simulink model "MagnetoShield_Calibration"  (R2019a)
settings: Solver=FixedStepAuto  StartTime=0.0  StopTime=10  RelTol=1e-3  EnableMultiTasking=on
libraries: arduinolib x1
settings Model: SimulationMode=external  ExtModeTrigDuration=2  Creator=Jakub  LastModifiedBy=Gergely
settings OptimizationCC: EnhancedBackFolding=on  PassReuseOutputArgsAs=Individual arguments  MaxStackSize=64  OptimizeBlockOrder=speed  DifferentSizesBufferReuse=on  OptimizationCustomize=off
settings DebuggingCC: ParameterTunabilityLossMsg=error
settings HardwareCC: ProdBitPerPointer=32  ProdBitPerSizeT=32  ProdBitPerPtrDiffT=32  ProdLargestAtomicInteger=Long  ProdLargestAtomicFloat=Double  ProdWordSize=32  ProdHWDeviceType=ARM Compatible->ARM Cortex
settings SFSimCC: MATLABDynamicMemAlloc=off
settings RTWCC: SystemTargetFile=ert.tlc  HardwareBoard=Arduino Due  TLCOptions=-aInlineSetEventsForThisBaseRateFcn=TLC_FALSE -aSuppressMultiTaskScheduler=TLC_FALSE -aRateBasedStepFcn=1  TemplateMakefile=ert_default_tmf  GenerateReport=on  Toolchain=Arduino ARM  BuildConfiguration=Faster Runs  IncludeHyperlinkInReport=on  LaunchReport=on  GenerateTraceInfo=on  GenerateTraceReport=on  GenerateTraceReportSl=on  GenerateTraceReportSf=on  GenerateTraceReportEml=on
settings CodeAppCC: ForceParamTrailComments=on  IgnoreCustomStorageClasses=off  OperatorAnnotations=on  SimulinkDataObjDesc=on  SFDataObjDesc=on  InsertBlockDesc=on
settings ERTTargetCC: SupportContinuousTime=on  SupportVariableSizeSignals=on  ExtModeStaticAllocSize=24576

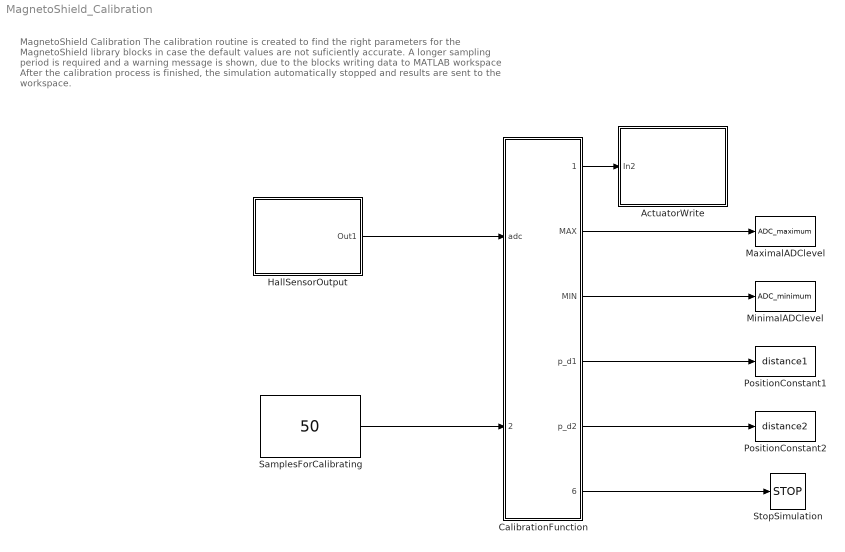
== system MagnetoShield_Calibration ==
  note: MagnetoShield Calibration
      | The calibration routine is created to find the right parameters for the MagnetoShield library blocks in case the default values are not suficiently accurate.
      |
      | A longer sampling period is required and a warning message is shown, due to the blocks writing data to MATLAB workspace
      |
      | After the calibration process is finished, the simulation automatically stopped and results are sent to the workspace.
  ActuatorWrite : Subsystem  AncestorBlock=MagnetoLibrary/ActuatoWrite  mask{Board=DUE, Units=Volts}
      mask prompts: Board "Type of the Arduino board"; Units "Input unite"
      mask help:
      | ActuatorWrite block allows to set desired voltage value on the electromagnet. The desired value can be expresed as voltage, percentage of maximal possible voltage or as a value of the magnetic field in Gausses as well.
      | This block converts input control signal into suficient form (16-bit number) and writes the information on the MCP4725-DAC converter.
      | Maximal voltage range: 0-12 V
      mask init:
      | mask_popup = get_param(gcb,'Board'); % which popup is choosen
      | % path to the I2C Write block
      | system = gcb;
      | way = strcat(system,'/I2C Write UNO');
      | % set Module based on Arduino type
      | if strcmp(mask_popup(1),'U')
      |     set_param(way,'I2CModule','0'); % Uno/Mega - module 0
      | elseif strcmp(mask_popup(1),'D')
      |     set_param(way,'I2CModule','1'); % Due - module 1
      | end
      settings: CopyFcn=set_param(gcb, 'LinkStatus', 'inactive')
      mask TypeOptions Board: UNO/MEGA | DUE
      mask TypeOptions Units: Volts | Percents | DAC levels
      mask DialogControl DescGroupVar Prompt: ActuatorWrite block
      mask Display: image('assets\MagnetoFig\ActuatorWrite.bmp');
  CalibrationFunction : MATLAB Function  TreatAsAtomicUnit=on
  HallSensorOutput : Subsystem  AncestorBlock=MagnetoLibrary/MagnetoShieldPins  mask{PIN=Hall sensor pin (A3), sampling=0.008}
      mask prompts: PIN "Choose pin"; sampling "Sampling period [s]"
      mask help:
      | User can choose a pin on which the data should be processed.
      | >Hall sensor pin - data about the possition of the levitating magnet.
      | >Voltage pin - voltage on the electromagnet
      | >Current pin - current crossing the electromagnet
      | >Reference pin - data from potentiometer, used as adjustable analog reference
      | (output = double)
      mask init:
      | letter = PIN;
      | if letter==1
      | path='assets\MagnetoFig\Pins\hpin.bmp';
      | elseif letter==2
      | path='assets\MagnetoFig\Pins\vpin.bmp';
      | elseif letter==3
      | path='assets\MagnetoFig\Pins\cpin.bmp';
      | else
      | path='assets\MagnetoFig\Pins\ppin.bmp';    
      | end
      settings: CopyFcn=set_param(gcb, 'LinkStatus', 'inactive')
      mask TypeOptions PIN: Hall sensor pin (A3) | Voltage pin (A1) | Current pin (A2) | Reference pin (A0)
      mask Callback PIN:
      | mask_popup = get_param(gcb,'PIN'); % which popup is choosen
      | % path to the I2C Write block
      | system = gcb;
      | way = strcat(system,'/Analog Input');
      | % set Module based on Arduino type
      | if strcmp(mask_popup(1),'H')
      |     set_param(way,'pinNumber','3'); % Uno/Mega - module 0
      | elseif strcmp(mask_popup(1),'V')
      |     set_param(way,'pinNumber','1'); % Due - module 1
      | elseif strcmp(mask_popup(1),'C')
      |     set_param(way,'pinNumber','2'); % Due - module 1
      | elseif strcmp(mask_popup(1),'R')
      |     set_param(way,'pinNumber','0'); % Due - module 11
      | end
      mask DialogControl DescGroupVar Prompt: MagnetoShieldPins block
      mask Display: image(path);
  MaximalADClevel : ToWorkspace  VariableName=ADC_maximum  SampleTime=-1
      settings: MaxDataPoints=1  Save2DSignal=2-D array (concatenate along first dimension)
  MinimalADClevel : ToWorkspace  VariableName=ADC_minimum  SampleTime=-1
      settings: MaxDataPoints=1  Save2DSignal=2-D array (concatenate along first dimension)
  PositionConstant1 : ToWorkspace  VariableName=distance1  SampleTime=-1
      settings: MaxDataPoints=1  Save2DSignal=2-D array (concatenate along first dimension)
  PositionConstant2 : ToWorkspace  VariableName=distance2  SampleTime=-1
      settings: MaxDataPoints=1  Save2DSignal=2-D array (concatenate along first dimension)
  SamplesForCalibrating : Constant  Value=50  SampleTime=0.008
  StopSimulation : Stop
  wires:
  CalibrationFunction/1(voltage) -> ActuatorWrite/1(In2)
  CalibrationFunction/2(MAX) -> MaximalADClevel/1
  CalibrationFunction/3(MIN) -> MinimalADClevel/1
  CalibrationFunction/6(terminate) -> StopSimulation/1
  HallSensorOutput/1(Out1) -> CalibrationFunction/1(adc)
  SamplesForCalibrating/1 -> CalibrationFunction/2(samples)
  CalibrationFunction/4(p_d1) -> PositionConstant1/1
  CalibrationFunction/5(p_d2) -> PositionConstant2/1

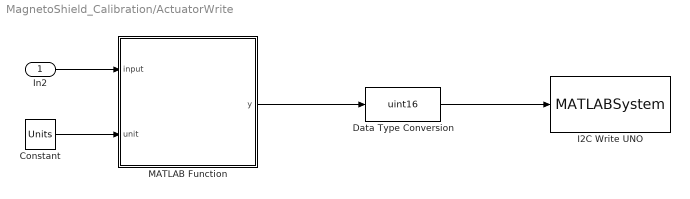
== system MagnetoShield_Calibration/ActuatorWrite ==
  In2 : Inport
  Constant : Constant  Value=Units
  Data Type Conversion : DataTypeConversion  OutDataTypeStr=uint16
  I2C Write UNO : MATLABSystem  AncestorBlock=arduinolib/I2C Write  InitFcn=|  System=codertarget.arduinobase.internal.arduinoI2CWrite  I2CModule=1  Mode=Master  SlaveAddress=96  SlaveByteOrder=BigEndian  Direction=Transmitter  RegisterAddressMode=off  RegisterAddress=0  SlaveDataType=uint8  DataLength=1  NoAck=off  RepeatedStart=off  OutputStatus=off  blockPlatform=ARDUINO
      | codertarget.arduinobase.blocks.registerI2CBlock(gcbh);
      | codertarget.arduinobase.blocks.arduinoBlockInitFcnCallback(gcbh);
      mask Type: I2C Write
      mask Display:
      | color('white');
      | plot([100,100,100,100],[100,100,100,100]);
      | plot([0,0,0,0],[0,0,0,0]);
      | color('blue');
      | text(99, 92, 'ARDUINO', 'horizontalAlignment', 'right');
      | color('black');
      | text(50,60,'\fontsize{12}\bfI2C','texmode','on','horizontalAlignment','center','verticalAlignment','middle');
      | text(50,40,'\fontsize{10}\bfMaster Write','texmode','on','horizontalAlignment','center','verticalAlignment','middle');
      | text(50,15,'Slave: 0x60' ,'horizontalAlignment', 'center');
      | port_label('input',1,'Data');
  MATLAB Function : MATLAB Function  TreatAsAtomicUnit=on
  wires:
  MATLAB Function/1(y) -> Data Type Conversion/1
  Data Type Conversion/1 -> I2C Write UNO/1
  Constant/1 -> MATLAB Function/2(unit)
  In2/1 -> MATLAB Function/1(input)

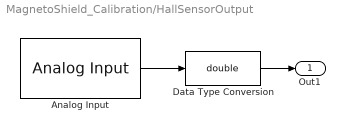
== system MagnetoShield_Calibration/HallSensorOutput ==
  Analog Input : arduinolib/Analog Input  pinNumber=3  ReadResultsOnly=off  ConversionTriggerSource=Software  ExternalTriggerType=uint32(0)  OutputDataType=uint16  EnableConversionCompleteNotify=off  EnableOuputStatus=off  SampleTime=sampling  blockPlatform=arduino
  Data Type Conversion : DataTypeConversion  OutDataTypeStr=double
  Out1 : Outport
  wires:
  Data Type Conversion/1 -> Out1/1
  Analog Input/1 -> Data Type Conversion/1

== matlab function MagnetoShield_Calibration/CalibrationFunction ==
  data: adc input; voltage output; samples input; MAX output; MIN output; p_d1 output; p_d2 output; terminate output
function [voltage,MAX,MIN,p_d1,p_d2,terminate]  = fcn(adc,samples)
persistent adcMAX adcMIN counter;
terminate = 0;

if isempty(counter) % inital values of extremes and the counter
    counter = 0;
    adcMAX = 300;
    adcMIN = 300;
end

% Minimal ADC level measured on the hall sensor
if counter<=samples
    voltage = 0;
    if adc<adcMIN
        adcMIN = adc;
    end
     MIN = 0;        % outputs of the function during data collection
     MAX = 0;
     p_d1 = 0;
     p_d2 = 0;
% Maximal ADC level measured on the hall sensor
elseif counter>samples && counter<=(2*samples)
    voltage = 12;
    if adc>adcMAX
        adcMAX = adc; 
    end
    MIN = 0;
    MAX = 0;
    p_d1 = 0;
    p_d2 = 0;
% Postprocessing of the measured data and termination of the simulation
else
    voltage = 0;    % Return magnet to the initial position        
    MAX = adcMAX;   % Extrems of ADC levels
    MIN = adcMIN;
    % Constants for position computation in [mm]
    p_d2 = log(17/12)/log((2.5-adcMIN*3.3/4095)*769.23/((2.5-adcMAX*3.3/4095)*769.23));
    p_d1 = 12/((2.5-adcMAX*3.3/4095)*769.23)^p_d2;
    terminate= 1; % terminate simulation
end

counter = counter+1;
end

== matlab function MagnetoShield_Calibration/ActuatorWrite/MATLAB Function ==
  data: input input; y output; unit input
function y = fcn(input,unit)

if unit==1 % voltage
    y = 4095/12*input;
elseif unit==2 % percents
    y = 4095/100*input;
elseif unit==3 % dac levels
    y = input;
else
     y = 0; % needed instance
end
% secures that 12-bit number will not overcross a size boundary
if y>4095
    y=4095;
elseif y<0
    y=0;
end

end
